simulink model "walkingRobotOptim"  (R2024b)
settings: Solver=ode15s  StartTime=0.0  StopTime=10  EnableMultiTasking=on
PreLoadFcn:
  | robotParameters
  | 
  | % Trajectory sample time
  | tsTraj = 0.01;
  | 
  | % Simulate air drag for stability
  | world_damping = 20; % Translational damping
  | world_rot_damping = 10;  % Rotational damping
  | 
  | % Only run if CAD model has changed on OnShape
  | %run("OnshapeTest\Onshape_Test.m")
  | run("OnshapeTest\Assembly1_DataFile.m")
InitFcn:
  |     % Evaluate the trajectory at the start and halfway points for right and
  |     % left legs, respectively, to get initial conditions and trajectory
  |     % waypoint derivatives
  |     [q_F,hip_der_F,knee_der_F] = createSmoothTrajectory( ...
  |         hip_motion_F,knee_motion_F,gait_period,[0 gait_period/2]);
  |     % Package up the initial conditions, keeping the yaw/roll joints fixed
  |     init_angs_FR = [-q_F(1,1) -q_F(2,1)];
  |     init_angs_FL = [-q_F(1,2) -q_F(2,2)];
  | 
  |     [q_H,hip_der_H,knee_der_H] = createSmoothTrajectory( ...
  |         hip_motion_H,knee_motion_H,gait_period,[0 gait_period/2]);
  |     % Package up the initial conditions, keeping the yaw/roll joints fixed
  |     init_angs_HR = [-q_H(1,1) -q_H(2,1)];
  |     init_angs_HL = [-q_H(1,2) -q_H(2,2)];
values from neighbouring files (symbols this model uses):
  gait_period = 2.5    [optimizedData_06Dec24_1101.mat]
  hip_der = [0, 0.5*( diff(hip(1:end-1)) + diff(hip(2:end)) )/dt, 0]    [createSmoothTrajectory.m]
  hip_motion_F = [-0.788016157275 -1.71688038519 -1.07878801066 0.273318560862 -0.349065850399]    [cheetah_waypoints.mat]    (also in optimizedData_06Dec24_1101.mat = [0.00380771774733 0.00304617419787 0.000761543549467 -0.0045; simulateWalkingRobot.m = deg2rad([params(1:N), params(1)]); walking_waypoints.mat = [-0.617466438509 -0.382533561491 0.182533561491 -0.382533561)
  hip_motion_H = [-0.350287580875 -0.0639663170856 1.07512281923 1.78425009431 0.280474410795]    [cheetah_waypoints.mat]    (also in optimizedData_06Dec24_1101.mat = [-0.0297001984292 0.827036294721 -0.277963395555 0.274155677; simulateWalkingRobot.m = deg2rad([params(2*N+1:3*N), params(2*N+1)]); walking_waypoints.mat = [-0.162257957554 -0.481537983524 -0.286227619971 0.130023561)
  knee_der = [0, 0.5*( diff(knee(1:end-1)) + diff(knee(2:end)) )/dt, 0]    [createSmoothTrajectory.m]
  knee_motion_F = [-0.479791011373 -1.75833195492 -2.37556764489 -1.2809844045 -0.532499954783]    [cheetah_waypoints.mat]    (also in optimizedData_06Dec24_1101.mat = [0.011423153242 0.0144693274399 0.0137077838904 0.0129462403; simulateWalkingRobot.m = deg2rad([params(N+1:2*N), params(N+1)]); walking_waypoints.mat = [0.119729530542 0.911553841048 0.391887203398 0.376829425011)
  knee_motion_H = [0.760789020944 2.09910749137 2.35340196339 1.93007235332 0.791332282854]    [cheetah_waypoints.mat]    (also in optimizedData_06Dec24_1101.mat = [-0.34269459726 -0.132508577607 -0.389148753778 0.1713472986; simulateWalkingRobot.m = deg2rad([params(3*N+1:4*N), params(3*N+1)]); walking_waypoints.mat = [0.397308136111 0.290525222789 0.655140986828 0.257025654272)
  N = numel(params)/4    [simulateWalkingRobot.m]
  traj_times = [0 0.25 0.5 0.75 1]    [cheetah_waypoints.mat]    (also in createSmoothTrajectory.m = linspace(0,period,numPoints); optimizedData_06Dec24_1101.mat = [0 0.5 1 1.5 2 2.5]; simulateWalkingRobot.m = linspace(0,gait_period,N+1); walking_waypoints.mat)
undefined symbols (not defined in the file or in its folder): ankle_der, back_leg_weight, body_weight, gravity, half_leg_weight, hip_der_F, hip_der_H, init_angs_R, knee_der_F, knee_der_H, plane_z, smiData, X, Y, Z
libraries: sm_lib x46, walkingRobotUtils x13, nesl_utility x4, robotcorelib x4, simulink x2
(part 1 of 2)
settings Model: SimulationMode=accelerator  Creator=bkim  LastModifiedBy=Andrew
settings SolverCC: AlgebraicLoopSolver=TrustRegion
settings DataIOCC: ReturnWorkspaceOutputs=off  OutputSaveName=simout  OutputTimes=0:0.01:10
settings OptimizationCC: LifeSpan=inf
settings DebuggingCC: UnconnectedInputMsg=warning  UnconnectedOutputMsg=warning  UnconnectedLineMsg=warning  AllowSymbolicDim=off  PregeneratedLibrarySubsystemCodeDiagnostic=none  SFUnexpectedBacktrackingDiag=warning  SFNoUnconditionalDefaultTransitionDiag=warning  SFExecutionAtInitializationDiag=none  UnitsInconsistencyMsg=none  ArithmeticOperatorsInVariantConditions=warning
settings ModelReferenceCC: EnableRefExpFcnMdlSchedulingChecks=on
settings SFSimCC: SimUseLocalCustomCode=off  CustomCodeUndefinedFunction=UseInterfaceOnly
settings RTWCC: RTWUseLocalCustomCode=off  GPUComputeCapability=3.5
settings CodeAppCC: StateflowObjectComments=on
settings GRTTargetCC: TargetLangStandard=C89/C90 (ANSI)
settings ConfigComp: CovMetricSettings=dw  CovSaveCumulativeToWorkspaceVar=on  CovSaveSingleToWorkspaceVar=on  CovExternalEMLEnable=off  CovSFcnEnable=off
settings SimscapeCC: SimscapeNormalizeSystem=off  SimscapeLogOpenViewer=on  SimscapeLogLimitData=off  SimscapeLogDataHistory=10000
settings ConfigurationSet: Description=SimMechanics 2G
settings DiagnosticsConfigSet: SimMechanicsRigidlyBoundBlock=none
settings ExplorerConfigSet: SimMechanicsOpenEditorOnUpdate=off  InternalSimMechanicsExplorerSettings="<ExplorerConfiguration><canonicalview>default</canonicalview><AnimationSetting><BasePlaybackSpeed>1.0</BasePlaybackSpeed><PlaybackSpeedFactor>1.0</PlaybackSpeedFactor></AnimationSetting><TilePanel><TileInfo><Tiles Columns=\"1\" Count=\"1\" Rows=\"1\"><Column Weight=\"1\"/><Row Weight=\"1\"/><Tile Height=\"1\" Width=\"1\" X=\"0\" Y=\"0\"/></Tiles></TileInfo><SceneInfo><SceneViewer><BGColor><R>0.60000002384185791</R><G>0.60000002384185791</G><B>0.60000002384185791</B></BGColor><Camera><DoPerspective>off</DoPerspective><Position><X>-6.96629667239135308</X><Y>24.6054722866086557</Y><Z>5.12968018743748999</Z></Position><Center><X>2.4732135105562727</X><Y>-3.90012739093662164</Y><Z>-2.29509835736230228</Z></Center><Up><X>0.317576681516579584</X><Y>-0.139145800878009762</Y><Z>0.937967748621952424</Z></Up><ViewLimDist>1</ViewLimDist><YLim>3.00115752214017162</YLim><XLim>3.84407522125978751</XLim></Camera></SceneViewer></SceneInfo></TilePanel><MechEditorPanel><Cameras/><GfxPanelCameraMap/><VideoCreator><PlaybackSpeedRatio>1.0</PlaybackSpeedRatio><FrameRate>30</FrameRate><VideoFormat>Motion JPEG AVI</VideoFormat><FrameSize>auto</FrameSize></VideoCreator></MechEditorPanel></ExplorerConfiguration>"

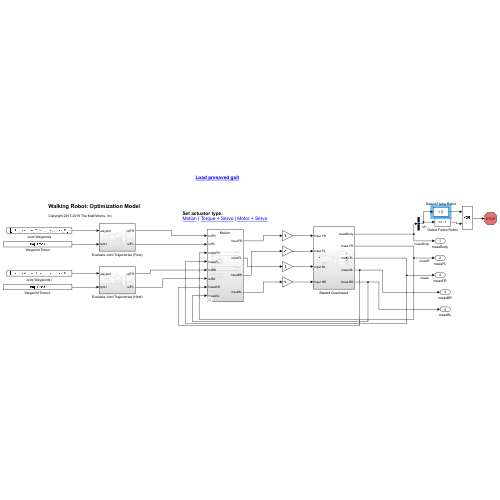
[thumbnail: Simulink's stored preview of the top-level diagram]
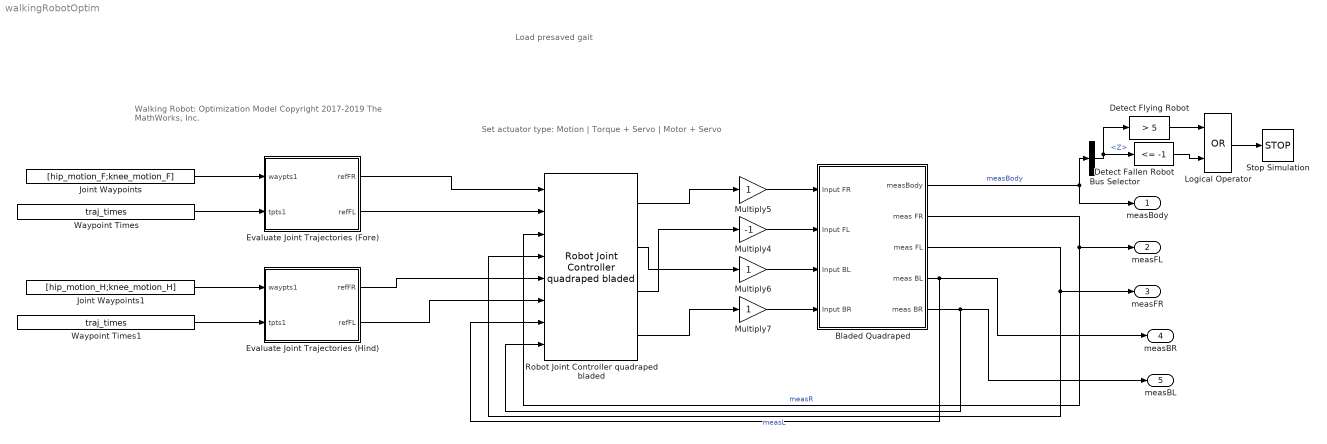
== system walkingRobotOptim ==
  note: Load presaved gait
  note: Walking Robot: Optimization Model
      |
      | Copyright 2017-2019 The MathWorks, Inc.
  note: Set actuator type:
      | Motion | Torque + Servo | Motor + Servo
  Bladed Quadraped : Subsystem
  Bus Selector : BusSelector  OutputSignals=Z
  Detect Fallen Robot : simulink/Logic and Bit Operations/Compare To Constant  relop=<=  const=-1  OutDataTypeStr=boolean
  Detect Flying Robot : simulink/Logic and Bit Operations/Compare To Constant  relop=>  const=5  OutDataTypeStr=boolean
  Evaluate Joint Trajectories (Fore) : Subsystem
  Evaluate Joint Trajectories (Hind) : Subsystem
  Joint Waypoints : Constant  Value=[hip_motion_F;knee_motion_F]
  Joint Waypoints1 : Constant  Value=[hip_motion_H;knee_motion_H]
  Logical Operator : Logic  Operator=OR  AllPortsSameDT=off  OutDataTypeStr=boolean
  Multiply4 : Gain  Gain=-1
  Multiply5 : Gain
  Multiply6 : Gain
  Multiply7 : Gain
  Robot Joint Controller quadraped bladed : walkingRobotUtils/Robot Joint Controller quadraped bladed  SystemSampleTime=-1  VariantActivationTime=update diagram  AllowFlexibleInterface=on  Latency=0  AutoFrameSizeCalculation=off
  Stop Simulation : Stop
  Waypoint Times : Constant  Value=traj_times
  Waypoint Times1 : Constant  Value=traj_times
  measBody : Outport  VectorParamsAs1DForOutWhenUnconnected=off
  measFL : Outport  Port=2  VectorParamsAs1DForOutWhenUnconnected=off
  measFR : Outport  Port=3  VectorParamsAs1DForOutWhenUnconnected=off
  measBR : Outport  Port=4  VectorParamsAs1DForOutWhenUnconnected=off
  measBL : Outport  Port=5  VectorParamsAs1DForOutWhenUnconnected=off
  wires:
  Bladed Quadraped/3(meas FL) -> Robot Joint Controller quadraped bladed/4, measFR/1  "measL"
  Bladed Quadraped/2(meas FR) -> Robot Joint Controller quadraped bladed/3, measFL/1  "measR"
  Bladed Quadraped/1(measBody) -> measBody/1, Bus Selector/1  "measBody"
  Bus Selector/1 -> Detect Flying Robot/1, Detect Fallen Robot/1  "<Z>"
  Detect Fallen Robot/1 -> Logical Operator/2
  Logical Operator/1 -> Stop Simulation/1
  Detect Flying Robot/1 -> Logical Operator/1
  Bladed Quadraped/4(meas BL) -> Robot Joint Controller quadraped bladed/7, measBR/1
  Bladed Quadraped/5(meas BR) -> Robot Joint Controller quadraped bladed/8, measBL/1
  Joint Waypoints/1 -> Evaluate Joint Trajectories (Fore)/1(waypts1)
  Evaluate Joint Trajectories (Fore)/1(refFR) -> Robot Joint Controller quadraped bladed/1
  Waypoint Times/1 -> Evaluate Joint Trajectories (Fore)/2(tpts1)
  Robot Joint Controller quadraped bladed/1 -> Multiply5/1
  Multiply6/1 -> Bladed Quadraped/3(Input BL)
  Robot Joint Controller quadraped bladed/4 -> Multiply7/1
  Multiply5/1 -> Bladed Quadraped/1(Input FR)
  Multiply7/1 -> Bladed Quadraped/4(Input BR)
  Robot Joint Controller quadraped bladed/2 -> Multiply6/1
  Multiply4/1 -> Bladed Quadraped/2(Input FL)
  Robot Joint Controller quadraped bladed/3 -> Multiply4/1
  Evaluate Joint Trajectories (Fore)/2(refFL) -> Robot Joint Controller quadraped bladed/2
  Evaluate Joint Trajectories (Hind)/1(refFR) -> Robot Joint Controller quadraped bladed/5
  Waypoint Times1/1 -> Evaluate Joint Trajectories (Hind)/2(tpts1)
  Joint Waypoints1/1 -> Evaluate Joint Trajectories (Hind)/1(waypts1)
  Evaluate Joint Trajectories (Hind)/2(refFL) -> Robot Joint Controller quadraped bladed/6

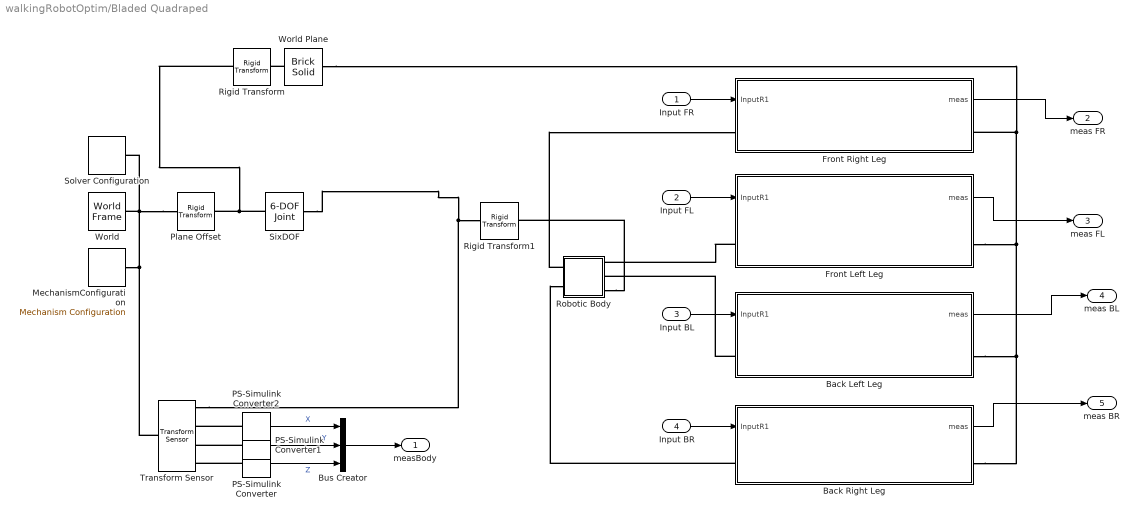
== system walkingRobotOptim/Bladed Quadraped ==
  Input FR : Inport
  Input FL : Inport  Port=2
  Input BL : Inport  Port=3
  Input BR : Inport  Port=4
  Back Left Leg : Subsystem
  Back Right Leg : Subsystem
  Bus Creator : BusCreator  Inputs=3
  Front Left Leg : Subsystem
  Front Right Leg : Subsystem
  MechanismConfiguration : sm_lib/Utilities/Mechanism Configuration  UniformGravity=Constant  GravityVector="[0 0  -gravity]"  GravityVectorUnits=m/s^2  LinearizationDelta=0.001  JointModeTransitionNonlinearIterations=2
  PS-Simulink Converter : nesl_utility/PS-Simulink Converter  PhysicalDomain=network_engine_domain  SubClassName=ps_output  LeftPortType=input  RightPortType=output  PseudoPeriodic=off  Frequencies=[]  VectorFormat=1-D array  Unit=m  AffineConversion=off
  PS-Simulink Converter1 : nesl_utility/PS-Simulink Converter  PhysicalDomain=network_engine_domain  SubClassName=ps_output  LeftPortType=input  RightPortType=output  PseudoPeriodic=off  Frequencies=[]  VectorFormat=1-D array  Unit=m  AffineConversion=off
  PS-Simulink Converter2 : nesl_utility/PS-Simulink Converter  PhysicalDomain=network_engine_domain  SubClassName=ps_output  LeftPortType=input  RightPortType=output  PseudoPeriodic=off  Frequencies=[]  VectorFormat=1-D array  Unit=m  AffineConversion=off
  Plane Offset : sm_lib/Frames and Transforms/Rigid Transform  RotationMethod=ArbitraryAxis  FollAlignAxisA=+X  BaseAlignAxisA=+Y  FollAlignAxisB=+Y  BaseAlignAxisB=+Z  RotationStandardAxis=+Z  RotationAngle=smiData.RigidTransform(17).angle  RotationAngleUnits=rad  RotationArbitraryAxis=smiData.RigidTransform(17).axis  RotationSequenceAxes=FollowerAxes  RotationSequence=XYX  RotationSequenceAngles=[0 0 0]  RotationSequenceAnglesUnits=deg  RotationMatrix=[1 0 0;0 1 0;0 0 1]  Quaternion=[1 0 0 0]  TranslationMethod=Cartesian  TranslationCartesianOffset=smiData.RigidTransform(17).translation  TranslationCartesianOffsetUnits=mm  TranslationStandardAxis=+Z  TranslationStandardOffset=0  TranslationStandardOffsetUnits=m  TranslationROffset=0  TranslationROffsetUnits=m  TranslationThetaOffset=0  TranslationThetaOffsetUnits=deg  TranslationZOffset=0  TranslationZOffsetUnits=m
  Rigid Transform : sm_lib/Frames and Transforms/Rigid Transform  RotationMethod=StandardAxis  FollAlignAxisA=+X  BaseAlignAxisA=+Y  FollAlignAxisB=+Y  BaseAlignAxisB=+Z  RotationStandardAxis=+Z  RotationAngle=90  RotationAngleUnits=deg  RotationArbitraryAxis=[0 0 1]  RotationSequenceAxes=FollowerAxes  RotationSequence=XYX  RotationSequenceAngles=[0 0 0]  RotationSequenceAnglesUnits=deg  RotationMatrix=[1 0 0;0 1 0;0 0 1]  Quaternion=[1 0 0 0]  TranslationMethod=StandardAxis  TranslationCartesianOffset=[0 0 0]  TranslationCartesianOffsetUnits=m  TranslationStandardAxis=+Z  TranslationStandardOffset=1  TranslationStandardOffsetUnits=m  TranslationROffset=0  TranslationROffsetUnits=m  TranslationThetaOffset=0  TranslationThetaOffsetUnits=deg  TranslationZOffset=0  TranslationZOffsetUnits=m
  Rigid Transform1 : sm_lib/Frames and Transforms/Rigid Transform  RotationMethod=StandardAxis  FollAlignAxisA=+X  BaseAlignAxisA=+Y  FollAlignAxisB=+Y  BaseAlignAxisB=+Z  RotationStandardAxis=-X  RotationAngle=180  RotationAngleUnits=deg  RotationArbitraryAxis=[0 0 1]  RotationSequenceAxes=FollowerAxes  RotationSequence=XYX  RotationSequenceAngles=[0 0 0]  RotationSequenceAnglesUnits=deg  RotationMatrix=[1 0 0;0 1 0;0 0 1]  Quaternion=[1 0 0 0]  TranslationMethod=None  TranslationCartesianOffset=[0 0 0]  TranslationCartesianOffsetUnits=m  TranslationStandardAxis=+Z  TranslationStandardOffset=1.5  TranslationStandardOffsetUnits=m  TranslationROffset=0  TranslationROffsetUnits=m  TranslationThetaOffset=0  TranslationThetaOffsetUnits=deg  TranslationZOffset=0  TranslationZOffsetUnits=m
  Robotic Body : Subsystem
  SixDOF : sm_lib/Joints/6-DOF Joint  JointMode=Normal  CompositeWrenchDir=FollowerOnBase  CompositeWrenchFrame=BaseFrame  SenseConstraintForce=off  SenseConstraintTorque=off  SenseTotalForce=off  SenseTotalTorque=off  PxPositionTargetSpecify=off  PxPositionTargetPriority=High  PxPositionTargetValue=0  PxPositionTargetValueUnits=m  PxVelocityTargetSpecify=off  PxVelocityTargetPriority=High  PxVelocityTargetValue=0  PxVelocityTargetValueUnits=m/s  PxEquilibriumPosition=0  PxEquilibriumPositionUnits=m  PxSpringStiffness=0  PxSpringStiffnessUnits=N/m  PxDampingCoefficient=0  PxDampingCoefficientUnits=N/(m/s)  PxLowerLimitSpecify=off  PxLowerLimitBound=-1  PxLowerLimitBoundUnits=m  PxLowerLimitStiffness=1e6  PxLowerLimitStiffnessUnits=N/m  PxLowerLimitDamping=1e3  PxLowerLimitDampingUnits=N/(m/s)  PxLowerLimitTransitionRegionWidth=1e-4  PxLowerLimitTransitionRegionWidthUnits=m  PxUpperLimitSpecify=off  PxUpperLimitBound=1  PxUpperLimitBoundUnits=m  PxUpperLimitStiffness=1e6  PxUpperLimitStiffnessUnits=N/m  PxUpperLimitDamping=1e3  PxUpperLimitDampingUnits=N/(m/s)  PxUpperLimitTransitionRegionWidth=1e-4  PxUpperLimitTransitionRegionWidthUnits=m  PxTorqueActuationMode=NoTorque  PxMotionActuationMode=ComputedMotion  PxSensePosition=off  PxSenseVelocity=off  PxSenseAcceleration=off  PxSenseTorqueForce=off  PxSenseLowerLimitTorqueForce=off  PxSenseUpperLimitTorqueForce=off  PyPositionTargetSpecify=off  PyPositionTargetPriority=High  PyPositionTargetValue=0  PyPositionTargetValueUnits=m  PyVelocityTargetSpecify=off  PyVelocityTargetPriority=High  PyVelocityTargetValue=0  PyVelocityTargetValueUnits=m/s  PyEquilibriumPosition=0  PyEquilibriumPositionUnits=m  PySpringStiffness=0  PySpringStiffnessUnits=N/m  PyDampingCoefficient=0  PyDampingCoefficientUnits=N/(m/s)  PyLowerLimitSpecify=off  PyLowerLimitBound=-1  PyLowerLimitBoundUnits=m  PyLowerLimitStiffness=1e6  PyLowerLimitStiffnessUnits=N/m  PyLowerLimitDamping=1e3  PyLowerLimitDampingUnits=N/(m/s)  PyLowerLimitTransitionRegionWidth=1e-4  PyLowerLimitTransitionRegionWidthUnits=m  PyUpperLimitSpecify=off  PyUpperLimitBound=1  PyUpperLimitBoundUnits=m  PyUpperLimitStiffness=1e6  PyUpperLimitStiffnessUnits=N/m  PyUpperLimitDamping=1e3  PyUpperLimitDampingUnits=N/(m/s)  PyUpperLimitTransitionRegionWidth=1e-4  PyUpperLimitTransitionRegionWidthUnits=m  PyTorqueActuationMode=NoTorque  PyMotionActuationMode=ComputedMotion  PySensePosition=off  PySenseVelocity=off  PySenseAcceleration=off  PySenseTorqueForce=off  PySenseLowerLimitTorqueForce=off  PySenseUpperLimitTorqueForce=off  PzPositionTargetSpecify=off  PzPositionTargetPriority=High  PzPositionTargetValue=0  PzPositionTargetValueUnits=m  PzVelocityTargetSpecify=off  PzVelocityTargetPriority=High  PzVelocityTargetValue=0  PzVelocityTargetValueUnits=m/s  PzEquilibriumPosition=0  PzEquilibriumPositionUnits=m  PzSpringStiffness=0  PzSpringStiffnessUnits=N/m  PzDampingCoefficient=0  PzDampingCoefficientUnits=N/(m/s)  PzLowerLimitSpecify=off  PzLowerLimitBound=-1  PzLowerLimitBoundUnits=m  PzLowerLimitStiffness=1e6  PzLowerLimitStiffnessUnits=N/m  PzLowerLimitDamping=1e3  PzLowerLimitDampingUnits=N/(m/s)  PzLowerLimitTransitionRegionWidth=1e-4  PzLowerLimitTransitionRegionWidthUnits=m  PzUpperLimitSpecify=off  PzUpperLimitBound=1  PzUpperLimitBoundUnits=m  PzUpperLimitStiffness=1e6  PzUpperLimitStiffnessUnits=N/m  PzUpperLimitDamping=1e3  PzUpperLimitDampingUnits=N/(m/s)  PzUpperLimitTransitionRegionWidth=1e-4  PzUpperLimitTransitionRegionWidthUnits=m  PzTorqueActuationMode=NoTorque  PzMotionActuationMode=ComputedMotion  PzSensePosition=off  PzSenseVelocity=off  PzSenseAcceleration=off  PzSenseTorqueForce=off  PzSenseLowerLimitTorqueForce=off  PzSenseUpperLimitTorqueForce=off  SphPositionTargetSpecify=off  SphPositionTargetPriority=High  SphPositionTargetRotationMethod=None  SphPositionTargetFollAlignAxisA=+X  SphPositionTargetBaseAlignAxisA=+Y  SphPositionTargetFollAlignAxisB=+Y  SphPositionTargetBaseAlignAxisB=+Z  SphPositionTargetRotationStandardAxis=+Z  SphPositionTargetRotationAngle=0  SphPositionTargetRotationAngleUnits=deg  SphPositionTargetRotationArbitraryAxis=[0 0 1]  SphPositionTargetRotationSequenceAxes=FollowerAxes  SphPositionTargetRotationSequence=XYX  SphPositionTargetRotationSequenceAngles=[0 0 0]  SphPositionTargetRotationSequenceAnglesUnits=deg  SphPositionTargetRotationMatrix=[1 0 0;0 1 0;0 0 1]  SphPositionTargetQuaternion=[1 0 0 0]  SphVelocityTargetSpecify=off  SphVelocityTargetPriority=High  SphVelocityTargetValue=[0 0 0]  SphVelocityTargetValueUnits=deg/s  SphVelocityTargetInFollowerFrame=on  SphEqPosRotationMethod=None  SphEqPosFollAlignAxisA=+X  SphEqPosBaseAlignAxisA=+Y  SphEqPosFollAlignAxisB=+Y  SphEqPosBaseAlignAxisB=+Z  SphEqPosRotationStandardAxis=+Z  SphEqPosRotationAngle=0  SphEqPosRotationAngleUnits=deg  SphEqPosRotationArbitraryAxis=[0 0 1]  SphEqPosRotationSequenceAxes=FollowerAxes  SphEqPosRotationSequence=XYX  SphEqPosRotationSequenceAngles=[0 0 0]  SphEqPosRotationSequenceAnglesUnits=deg  SphEqPosRotationMatrix=[1 0 0;0 1 0;0 0 1]  SphEqPosQuaternion=[1 0 0 0]  SphSpringStiffness=0  SphSpringStiffnessUnits=N*m/deg  SphDampingCoefficient=0  SphDampingCoefficientUnits=N*m/(deg/s)  SphLowerLimitSpecify=off  SphLowerLimitBound=15  SphLowerLimitBoundUnits=deg  SphLowerLimitStiffness=1e4  SphLowerLimitStiffnessUnits=N*m/deg  SphLowerLimitDamping=10  SphLowerLimitDampingUnits=N*m/(deg/s)  SphLowerLimitTransitionRegionWidth=0.1  SphLowerLimitTransitionRegionWidthUnits=deg  SphUpperLimitSpecify=off  SphUpperLimitBound=45  SphUpperLimitBoundUnits=deg  SphUpperLimitStiffness=1e4  SphUpperLimitStiffnessUnits=N*m/deg  SphUpperLimitDamping=10  SphUpperLimitDampingUnits=N*m/(deg/s)  SphUpperLimitTransitionRegionWidth=0.1  SphUpperLimitTransitionRegionWidthUnits=deg  SphTorqueActuationMode=NoTorque  SphActuateTorqueX=off  SphActuateTorqueY=off  SphActuateTorqueZ=off  SphActuateTorque=off  SphActuationFrame=BaseFrame  SphSensePosition=off  SphSenseVelocityX=off  SphSenseVelocityY=off  SphSenseVelocityZ=off  SphSenseVelocity=off  SphSenseAccelerationX=off  SphSenseAccelerationY=off  SphSenseAccelerationZ=off  SphSenseAcceleration=off  SphSenseLowerLimitTorqueMag=off  SphSenseUpperLimitTorqueMag=off  SphSensingFrame=FollowerFrame
  Solver Configuration : nesl_utility/Solver Configuration  PhysicalDomain=network_engine_domain  SubClassName=solver  LeftPortType=input  RightPortType=generic  Tones=[]  Harmonics=[]  SimulateNoise=off  Profile=off  UseLocalSampling=off  EnableSwitchedLinearOptims=on  FrequencyDomain=off  UseCCode=off  RelTol=0.001  AbsTol=0.001  MinStep=1e-09  ToWorkspace=off  RevertToSquareIcSolve=off  NumHomotopyIterations=100  PhasorMode=off  PhasorModeNumHarmonics=1  ConsistencySolver=NEWTON_XTOL_AFTER_FTOL  IndexReductionMethod=DerivativeReplacement  DoDC=off  ResidualTolerance=1e-09  ConsistencyTolSource=GLOBAL  ConsistencyAbsTol=0.001  ConsistencyRelTol=0.001  ConsistencyTolFactor=0.001  UseLocalSolver=off  LocalSolverChoice=NE_BACKWARD_EULER_ADVANCER  ResolveIndetEquations=on  FunctionEvalNumThread=1  LocalSolverSampleTime=0.001  DoFixedCost=off  MaxNonlinIter=3  MaxModeIter=2  ComputeImpulses=off  ImpulseIterations=2  LinearAlgebra=auto  LinearAlgebraNumThread=0  EquationFormulation=NE_TIME_EF  DelaysMemoryBudget=1024  AutomaticFiltering=on  FilteringTimeConstant=0.001  PartitionStorageMethod=AS_NEEDED  PartitionMemoryBudget=1024  PartitionMethod=ROBUST  MultibodyUseLocalSolver=off  MultibodyLocalSolverChoice=ODE1  MultibodyLocalSolverSampleTime=0.001
  Transform Sensor : sm_lib/Frames and Transforms/Transform Sensor  MeasurementFrame=World  RotationSequence=XYX  SenseAngle=off  SenseAxis=off  SenseQ=off  SenseR=off  SenseRotationSequence=off  SenseOmegaX=off  SenseOmegaY=off  SenseOmegaZ=off  SenseOmega=off  SenseQDot=off  SenseRDot=off  SenseRotationSequenceDot=off  SenseAlphaX=off  SenseAlphaY=off  SenseAlphaZ=off  SenseAlpha=off  SenseQDDot=off  SenseRDDot=off  SenseX=on  SenseY=on  SenseZ=on  SenseXYZ=off  SenseRad=off  SenseAzim=off  SenseDist=off  SenseInc=off  SenseXDot=off  SenseYDot=off  SenseZDot=off  SenseXYZDot=off  SenseRadDot=off  SenseAzimDot=off  SenseDistDot=off  SenseIncDot=off  SenseXDDot=off  SenseYDDot=off  SenseZDDot=off  SenseXYZDDot=off  SenseRadDDot=off  SenseAzimDDot=off  SenseDistDDot=off  SenseIncDDot=off
  World : sm_lib/Frames and Transforms/World Frame
  World Plane : sm_lib/Body Elements/Brick Solid  BrickDimensions=[100 100 plane_z]  BrickDimensionsUnits=m  ExportEntireGeometry=on  InertiaType=CalculateFromGeometry  BasedOnType=Density  Density=1000  DensityUnits=kg/(m^3)  Mass=1  MassUnits=kg  CenterOfMass=[0 0 0]  CenterOfMassUnits=m  MomentsOfInertia=[1 1 1]  MomentsOfInertiaUnits=kg*m^2  ProductsOfInertia=[0 0 0]  ProductsOfInertiaUnits=kg*m^2  GraphicType=FromGeometry  MarkerShape=Sphere  MarkerSize=10  GraphicVisPropType=SimpleVisualProperties  GraphicDiffuseColor=[0.6353 0.07843 0.1843]  GraphicOpacity=1  GraphicSpecularColor=[0.5 0.5 0.5 1.0]  GraphicAmbientColor=[0.15 0.15 0.15 1.0]  GraphicEmissiveColor=[0.0 0.0 0.0 1.0]  GraphicShininess=75  DoExposeReferenceFrame=on  SerializedFrames=<Frames/>
  measBody : Outport  VectorParamsAs1DForOutWhenUnconnected=off
  meas FR : Outport  Port=2  VectorParamsAs1DForOutWhenUnconnected=off
  meas FL : Outport  Port=3  VectorParamsAs1DForOutWhenUnconnected=off
  meas BL : Outport  Port=4  VectorParamsAs1DForOutWhenUnconnected=off
  meas BR : Outport  Port=5  VectorParamsAs1DForOutWhenUnconnected=off
  wires:
  PS-Simulink Converter1/1 -> Bus Creator/2  "Y"
  Bus Creator/1 -> measBody/1
  PS-Simulink Converter2/1 -> Bus Creator/1  "X"
  PS-Simulink Converter/1 -> Bus Creator/3  "Z"
  Input BR/1 -> Back Right Leg/1(InputR1)
  Front Right Leg/1(meas) -> meas FR/1
  Front Left Leg/1(meas) -> meas FL/1
  Back Left Leg/1(meas) -> meas BL/1
  Back Right Leg/1(meas) -> meas BR/1
  Input FL/1 -> Front Left Leg/1(InputR1)
  Input FR/1 -> Front Right Leg/1(InputR1)
  Input BL/1 -> Back Left Leg/1(InputR1)
  connections:
  Plane Offset/LConn1 -- Transform Sensor/LConn1 -- MechanismConfiguration/RConn1 -- Solver Configuration/RConn1 -- World/RConn1
  Back Left Leg/LConn1 -- Robotic Body/RConn2
  SixDOF/RConn1 -- Transform Sensor/RConn1 -- Rigid Transform1/LConn1
  Back Right Leg/LConn1 -- Robotic Body/LConn2
  Front Left Leg/LConn1 -- Robotic Body/RConn1
  PS-Simulink Converter1/LConn1 -- Transform Sensor/RConn3
  PS-Simulink Converter2/LConn1 -- Transform Sensor/RConn2
  PS-Simulink Converter/LConn1 -- Transform Sensor/RConn4
  World Plane/LConn1 -- Back Right Leg/RConn1 -- Back Left Leg/RConn1 -- Front Left Leg/RConn1 -- Front Right Leg/RConn1
  World Plane/RConn1 -- Rigid Transform/RConn1
  Plane Offset/RConn1 -- Rigid Transform/LConn1 -- SixDOF/LConn1
  Robotic Body/LConn1 -- Front Right Leg/LConn1
  Robotic Body/RConn3 -- Rigid Transform1/RConn1

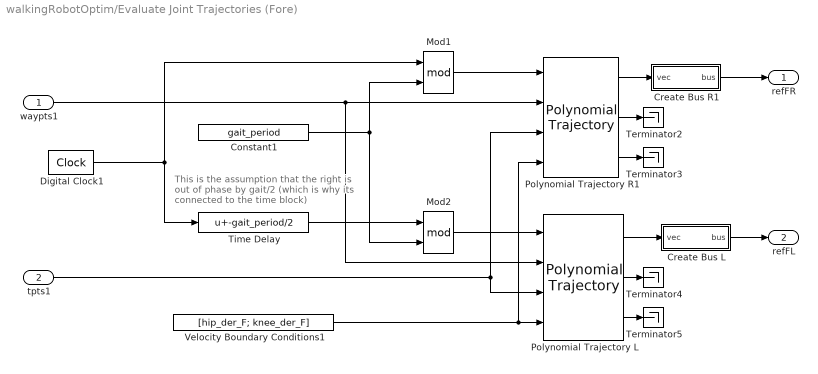
== system walkingRobotOptim/Evaluate Joint Trajectories (Fore) ==
  note: This is the assumption that the right is out of phase by gait/2 (which is why its connected to the time block)
  waypts1 : Inport
  tpts1 : Inport  Port=2
  Constant1 : Constant  Value=gait_period
  Create Bus L : Subsystem
  Create Bus R1 : Subsystem
  Digital Clock1 : DigitalClock  SampleTime=.01
  Mod1 : Math  Operator=mod
  Mod2 : Math  Operator=mod
  Polynomial Trajectory L : robotcorelib/Polynomial Trajectory  WaypointSource=External  Waypoints=[ 0, 2, 1, 5, 0; -1, 3, 1, 4, 4 ]  TimePoints=time  TimeInterval=[ 1, 4 ]  Method=Cubic Polynomial  ParameterSource=External  VelocityBoundaryCondition=[hip_der; knee_der; ankle_der]  AccelerationBoundaryCondition=zeros( 2, 5 )  SimulateUsing=Code generation
  Polynomial Trajectory R1 : robotcorelib/Polynomial Trajectory  WaypointSource=External  Waypoints=[ 0, 2, 1, 5, 0; -1, 3, 1, 4, 4 ]  TimePoints=time  TimeInterval=[ 1, 4 ]  Method=Cubic Polynomial  ParameterSource=External  VelocityBoundaryCondition=[hip_der; knee_der; ankle_der]  AccelerationBoundaryCondition=zeros( 2, 5 )  SimulateUsing=Code generation
  Terminator{2..5} (4 alike) : Terminator
  Time Delay : Bias  Bias=-gait_period/2  SaturateOnIntegerOverflow=off
  Velocity Boundary Conditions1 : Constant  Value=[hip_der_F; knee_der_F]
  refFR : Outport
  refFL : Outport  Port=2
  wires:
  Polynomial Trajectory L/3 -> Terminator5/1
  Velocity Boundary Conditions1/1 -> Polynomial Trajectory R1/4, Polynomial Trajectory L/4
  Create Bus L/1(bus) -> refFL/1
  Mod2/1 -> Polynomial Trajectory L/1
  Digital Clock1/1 -> Time Delay/1, Mod1/1
  Polynomial Trajectory R1/2 -> Terminator2/1
  tpts1/1 -> Polynomial Trajectory L/3, Polynomial Trajectory R1/3
  Polynomial Trajectory R1/3 -> Terminator3/1
  Polynomial Trajectory L/2 -> Terminator4/1
  Polynomial Trajectory R1/1 -> Create Bus R1/1(vec)
  waypts1/1 -> Polynomial Trajectory L/2, Polynomial Trajectory R1/2
  Mod1/1 -> Polynomial Trajectory R1/1
  Constant1/1 -> Mod1/2, Mod2/2
  Polynomial Trajectory L/1 -> Create Bus L/1(vec)
  Time Delay/1 -> Mod2/1
  Create Bus R1/1(bus) -> refFR/1

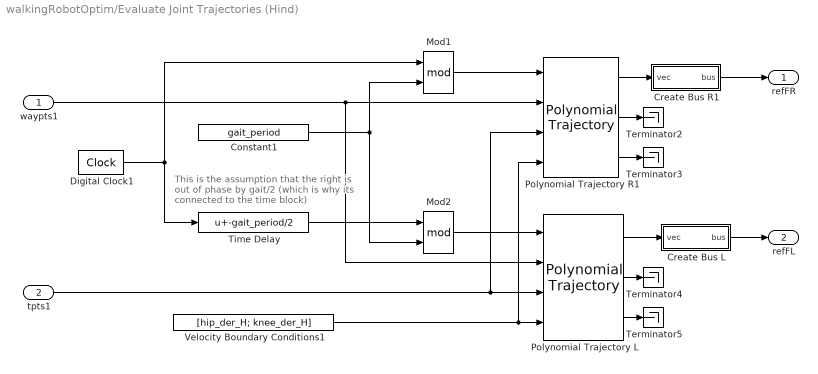
== system walkingRobotOptim/Evaluate Joint Trajectories (Hind) ==
  note: This is the assumption that the right is out of phase by gait/2 (which is why its connected to the time block)
  waypts1 : Inport
  tpts1 : Inport  Port=2
  Constant1 : Constant  Value=gait_period
  Create Bus L : Subsystem
  Create Bus R1 : Subsystem
  Digital Clock1 : DigitalClock  SampleTime=.01
  Mod1 : Math  Operator=mod
  Mod2 : Math  Operator=mod
  Polynomial Trajectory L : robotcorelib/Polynomial Trajectory  WaypointSource=External  Waypoints=[ 0, 2, 1, 5, 0; -1, 3, 1, 4, 4 ]  TimePoints=time  TimeInterval=[ 1, 4 ]  Method=Cubic Polynomial  ParameterSource=External  VelocityBoundaryCondition=[hip_der; knee_der; ankle_der]  AccelerationBoundaryCondition=zeros( 2, 5 )  SimulateUsing=Code generation
  Polynomial Trajectory R1 : robotcorelib/Polynomial Trajectory  WaypointSource=External  Waypoints=[ 0, 2, 1, 5, 0; -1, 3, 1, 4, 4 ]  TimePoints=time  TimeInterval=[ 1, 4 ]  Method=Cubic Polynomial  ParameterSource=External  VelocityBoundaryCondition=[hip_der; knee_der; ankle_der]  AccelerationBoundaryCondition=zeros( 2, 5 )  SimulateUsing=Code generation
  Terminator{2..5} (4 alike) : Terminator
  Time Delay : Bias  Bias=-gait_period/2  SaturateOnIntegerOverflow=off
  Velocity Boundary Conditions1 : Constant  Value=[hip_der_H; knee_der_H]
  refFR : Outport
  refFL : Outport  Port=2
  wires:
  Polynomial Trajectory L/3 -> Terminator5/1
  Velocity Boundary Conditions1/1 -> Polynomial Trajectory R1/4, Polynomial Trajectory L/4
  Create Bus L/1(bus) -> refFL/1
  Mod2/1 -> Polynomial Trajectory L/1
  Digital Clock1/1 -> Time Delay/1, Mod1/1
  Polynomial Trajectory R1/2 -> Terminator2/1
  tpts1/1 -> Polynomial Trajectory R1/3, Polynomial Trajectory L/3
  Polynomial Trajectory R1/3 -> Terminator3/1
  Polynomial Trajectory L/2 -> Terminator4/1
  Polynomial Trajectory R1/1 -> Create Bus R1/1(vec)
  waypts1/1 -> Polynomial Trajectory L/2, Polynomial Trajectory R1/2
  Mod1/1 -> Polynomial Trajectory R1/1
  Constant1/1 -> Mod1/2, Mod2/2
  Polynomial Trajectory L/1 -> Create Bus L/1(vec)
  Time Delay/1 -> Mod2/1
  Create Bus R1/1(bus) -> refFR/1

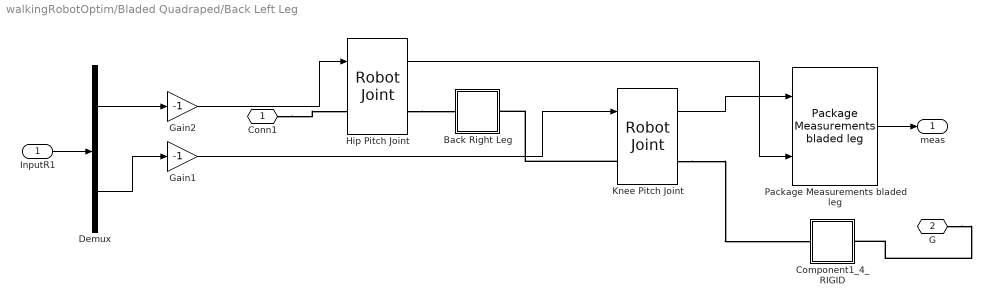
== system walkingRobotOptim/Bladed Quadraped/Back Left Leg ==
  InputR1 : Inport
  Back Right Leg : Subsystem
  Component1_4_RIGID : Subsystem
  Demux : Demux  Outputs=2
  Gain1 : Gain  Gain=-1
  Gain2 : Gain  Gain=-1
  Hip Pitch Joint : walkingRobotUtils/Robot Joint  jointDamping=joint_damping  initAngle=init_angs_HL(1)  upperLimit=pi/2  lowerLimit=-pi/2  limitK=1000  limitD=100
  Knee Pitch Joint : walkingRobotUtils/Robot Joint  jointDamping=joint_damping  initAngle=init_angs_HL(2)  upperLimit=pi/2  lowerLimit=-pi/2  limitK=1000  limitD=100
  Package Measurements bladed leg : walkingRobotUtils/Package Measurements bladed leg  SystemSampleTime=-1  VariantActivationTime=update diagram  AllowFlexibleInterface=on  Latency=0  AutoFrameSizeCalculation=off
  Conn1 : PMIOPort  Side=Left
  G : PMIOPort  Port=2  Side=Right
  meas : Outport  VectorParamsAs1DForOutWhenUnconnected=off
  wires:
  InputR1/1 -> Demux/1
  Gain1/1 -> Knee Pitch Joint/1
  Demux/2 -> Gain1/1
  Demux/1 -> Gain2/1
  Gain2/1 -> Hip Pitch Joint/1
  Hip Pitch Joint/1 -> Package Measurements bladed leg/2
  Knee Pitch Joint/1 -> Package Measurements bladed leg/1
  Package Measurements bladed leg/1 -> meas/1
  connections:
  Conn1/RConn1 -- Hip Pitch Joint/LConn1
  Knee Pitch Joint/RConn1 -- Component1_4_RIGID/LConn1
  G/RConn1 -- Component1_4_RIGID/RConn1
  Hip Pitch Joint/RConn1 -- Back Right Leg/LConn1
  Knee Pitch Joint/LConn1 -- Back Right Leg/RConn1

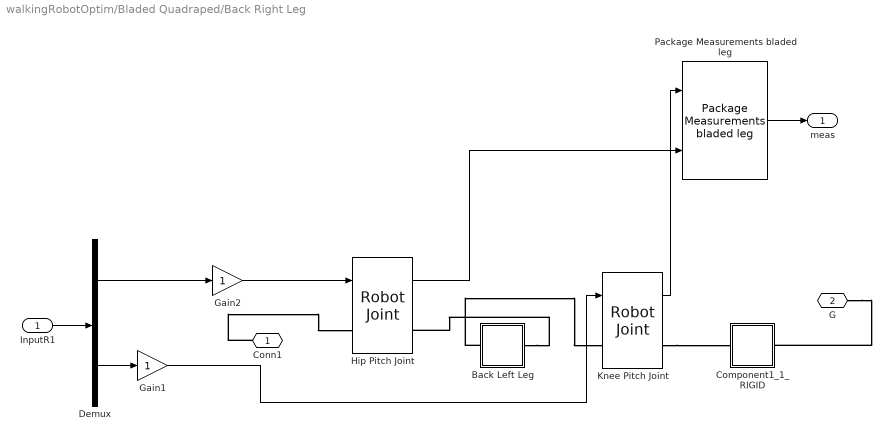
== system walkingRobotOptim/Bladed Quadraped/Back Right Leg ==
  InputR1 : Inport
  Back Left Leg : Subsystem
  Component1_1_RIGID : Subsystem
  Demux : Demux  Outputs=2
  Gain1 : Gain
  Gain2 : Gain
  Hip Pitch Joint : walkingRobotUtils/Robot Joint  jointDamping=joint_damping  initAngle=init_angs_HR(1)  upperLimit=pi/2  lowerLimit=-pi/2  limitK=1000  limitD=100
  Knee Pitch Joint : walkingRobotUtils/Robot Joint  jointDamping=joint_damping  initAngle=init_angs_HR(1)  upperLimit=pi/2  lowerLimit=-pi/2  limitK=1000  limitD=100
  Package Measurements bladed leg : walkingRobotUtils/Package Measurements bladed leg  SystemSampleTime=-1  VariantActivationTime=update diagram  AllowFlexibleInterface=on  Latency=0  AutoFrameSizeCalculation=off
  Conn1 : PMIOPort  Side=Left
  G : PMIOPort  Port=2  Side=Right
  meas : Outport  VectorParamsAs1DForOutWhenUnconnected=off
  wires:
  InputR1/1 -> Demux/1
  Demux/1 -> Gain2/1
  Demux/2 -> Gain1/1
  Hip Pitch Joint/1 -> Package Measurements bladed leg/2
  Package Measurements bladed leg/1 -> meas/1
  Knee Pitch Joint/1 -> Package Measurements bladed leg/1
  Gain2/1 -> Hip Pitch Joint/1
  Gain1/1 -> Knee Pitch Joint/1
  connections:
  G/RConn1 -- Component1_1_RIGID/RConn1
  Conn1/RConn1 -- Hip Pitch Joint/LConn1
  Knee Pitch Joint/RConn1 -- Component1_1_RIGID/LConn1
  Back Left Leg/RConn1 -- Hip Pitch Joint/RConn1
  Back Left Leg/LConn1 -- Knee Pitch Joint/LConn1

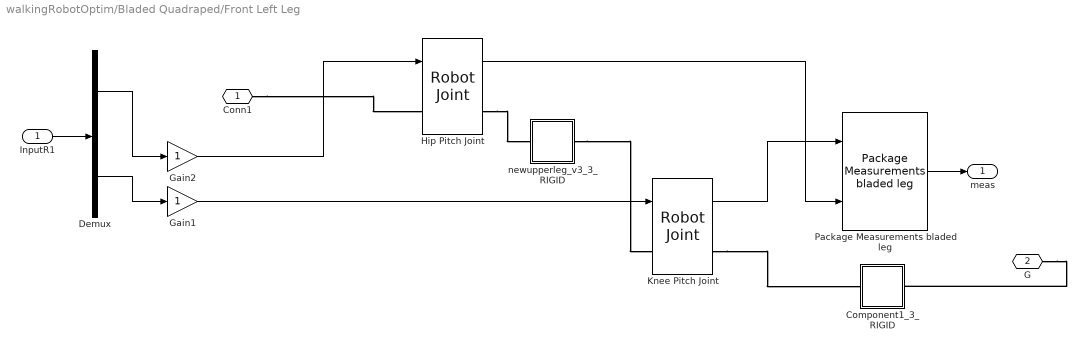
== system walkingRobotOptim/Bladed Quadraped/Front Left Leg ==
  InputR1 : Inport
  Component1_3_RIGID : Subsystem
  Demux : Demux  Outputs=2
  Gain1 : Gain
  Gain2 : Gain
  Hip Pitch Joint : walkingRobotUtils/Robot Joint  jointDamping=joint_damping  initAngle=init_angs_R(3)  upperLimit=pi/2  lowerLimit=-pi/2  limitK=1000  limitD=100
  Knee Pitch Joint : walkingRobotUtils/Robot Joint  jointDamping=joint_damping  initAngle=init_angs_R(5)  upperLimit=pi/2  lowerLimit=-pi/2  limitK=1000  limitD=100
  Package Measurements bladed leg : walkingRobotUtils/Package Measurements bladed leg  SystemSampleTime=-1  VariantActivationTime=update diagram  AllowFlexibleInterface=on  Latency=0  AutoFrameSizeCalculation=off
  newupperleg_v3_3_RIGID : Subsystem
  Conn1 : PMIOPort  Side=Left
  G : PMIOPort  Port=2  Side=Right
  meas : Outport  VectorParamsAs1DForOutWhenUnconnected=off
  wires:
  InputR1/1 -> Demux/1
  Demux/1 -> Gain2/1
  Demux/2 -> Gain1/1
  Gain2/1 -> Hip Pitch Joint/1
  Gain1/1 -> Knee Pitch Joint/1
  Hip Pitch Joint/1 -> Package Measurements bladed leg/2
  Knee Pitch Joint/1 -> Package Measurements bladed leg/1
  Package Measurements bladed leg/1 -> meas/1
  connections:
  G/RConn1 -- Component1_3_RIGID/RConn1
  Knee Pitch Joint/RConn1 -- Component1_3_RIGID/LConn1
  Conn1/RConn1 -- Hip Pitch Joint/LConn1
  Hip Pitch Joint/RConn1 -- newupperleg_v3_3_RIGID/LConn1
  newupperleg_v3_3_RIGID/RConn1 -- Knee Pitch Joint/LConn1

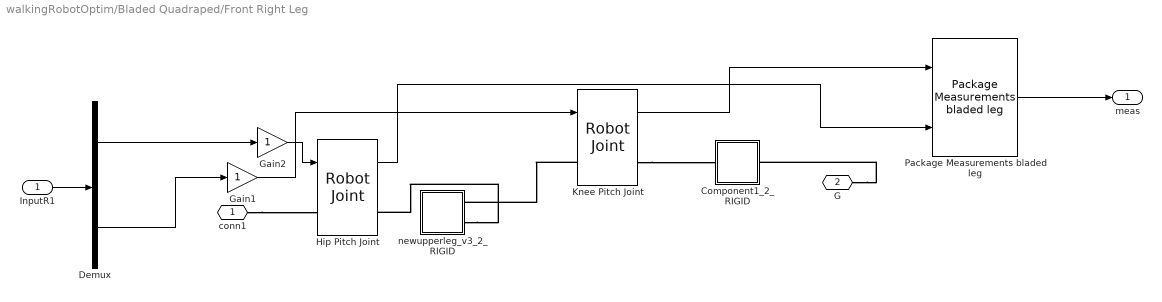
== system walkingRobotOptim/Bladed Quadraped/Front Right Leg ==
  InputR1 : Inport
  Component1_2_RIGID : Subsystem
  Demux : Demux  Outputs=2
  Gain1 : Gain
  Gain2 : Gain
  Hip Pitch Joint : walkingRobotUtils/Robot Joint  jointDamping=joint_damping  initAngle=init_angs_HR(1)  upperLimit=pi/2  lowerLimit=-pi/2  limitK=1000  limitD=100
  Knee Pitch Joint : walkingRobotUtils/Robot Joint  jointDamping=joint_damping  initAngle=init_angs_HR(2)  upperLimit=pi/2  lowerLimit=-pi/2  limitK=1000  limitD=100
  Package Measurements bladed leg : walkingRobotUtils/Package Measurements bladed leg  SystemSampleTime=-1  VariantActivationTime=update diagram  AllowFlexibleInterface=on  Latency=0  AutoFrameSizeCalculation=off
  newupperleg_v3_2_RIGID : Subsystem
  conn1 : PMIOPort  Side=Left
  G : PMIOPort  Port=2  Side=Right
  meas : Outport  VectorParamsAs1DForOutWhenUnconnected=off
  wires:
  Demux/2 -> Gain1/1
  InputR1/1 -> Demux/1
  Demux/1 -> Gain2/1
  Knee Pitch Joint/1 -> Package Measurements bladed leg/1
  Hip Pitch Joint/1 -> Package Measurements bladed leg/2
  Package Measurements bladed leg/1 -> meas/1
  Gain1/1 -> Knee Pitch Joint/1
  Gain2/1 -> Hip Pitch Joint/1
  connections:
  G/RConn1 -- Component1_2_RIGID/RConn1
  Knee Pitch Joint/RConn1 -- Component1_2_RIGID/LConn1
  Knee Pitch Joint/LConn1 -- newupperleg_v3_2_RIGID/RConn1
  conn1/RConn1 -- Hip Pitch Joint/LConn1
  newupperleg_v3_2_RIGID/RConn2 -- Hip Pitch Joint/RConn1

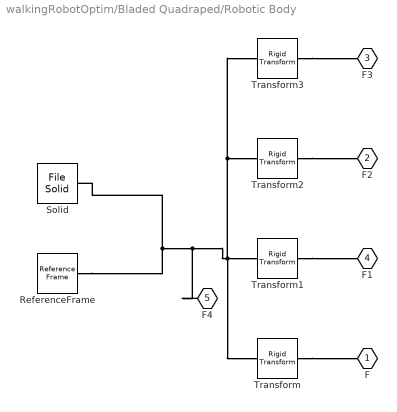
== system walkingRobotOptim/Bladed Quadraped/Robotic Body ==
  ReferenceFrame : sm_lib/Frames and Transforms/Reference Frame
  Solid : sm_lib/Body Elements/File Solid  ExtGeomFileName=robobody v1.step  UnitType=FromFile  ExtGeomFileUnits=m  StepReaderType=HEX  ExportConvexHullGeometry=off  InertiaType=CalculateFromGeometry  BasedOnType=Mass  Density=1000  DensityUnits=kg/m^3  Mass=body_weight  MassUnits=kg  CenterOfMass=smiData.Solid(3).CoM  CenterOfMassUnits=mm  MomentsOfInertia=smiData.Solid(3).MoI  MomentsOfInertiaUnits=lbm*mm^2  ProductsOfInertia=smiData.Solid(3).PoI  ProductsOfInertiaUnits=lbm*mm^2  GraphicType=FromGeometry  MarkerShape=Sphere  MarkerSize=10  GraphicVisPropType=SimpleVisualProperties  GraphicDiffuseColor=smiData.Solid(3).color  GraphicOpacity=smiData.Solid(3).opacity  GraphicSpecularColor=[0.5 0.5 0.5 1.0]  GraphicAmbientColor=[0.15 0.15 0.15 1.0]  GraphicEmissiveColor=[0.0 0.0 0.0 1.0]  GraphicShininess=75  DoExposeReferenceFrame=on  SerializedFrames=<Frames/>
  Transform : sm_lib/Frames and Transforms/Rigid Transform  RotationMethod=ArbitraryAxis  FollAlignAxisA=+X  BaseAlignAxisA=+Y  FollAlignAxisB=+Y  BaseAlignAxisB=+Z  RotationStandardAxis=+Z  RotationAngle=smiData.RigidTransform(2).angle  RotationAngleUnits=rad  RotationArbitraryAxis=smiData.RigidTransform(2).axis  RotationSequenceAxes=FollowerAxes  RotationSequence=XYX  RotationSequenceAngles=[0 0 0]  RotationSequenceAnglesUnits=deg  RotationMatrix=[1 0 0;0 1 0;0 0 1]  Quaternion=[1 0 0 0]  TranslationMethod=Cartesian  TranslationCartesianOffset=smiData.RigidTransform(2).translation  TranslationCartesianOffsetUnits=mm  TranslationStandardAxis=+Z  TranslationStandardOffset=0  TranslationStandardOffsetUnits=m  TranslationROffset=0  TranslationROffsetUnits=m  TranslationThetaOffset=0  TranslationThetaOffsetUnits=deg  TranslationZOffset=0  TranslationZOffsetUnits=m
  Transform1 : sm_lib/Frames and Transforms/Rigid Transform  RotationMethod=ArbitraryAxis  FollAlignAxisA=+X  BaseAlignAxisA=+Y  FollAlignAxisB=+Y  BaseAlignAxisB=+Z  RotationStandardAxis=+Z  RotationAngle=smiData.RigidTransform(7).angle  RotationAngleUnits=rad  RotationArbitraryAxis=smiData.RigidTransform(7).axis  RotationSequenceAxes=FollowerAxes  RotationSequence=XYX  RotationSequenceAngles=[0 0 0]  RotationSequenceAnglesUnits=deg  RotationMatrix=[1 0 0;0 1 0;0 0 1]  Quaternion=[1 0 0 0]  TranslationMethod=Cartesian  TranslationCartesianOffset=smiData.RigidTransform(7).translation  TranslationCartesianOffsetUnits=mm  TranslationStandardAxis=+Z  TranslationStandardOffset=0  TranslationStandardOffsetUnits=m  TranslationROffset=0  TranslationROffsetUnits=m  TranslationThetaOffset=0  TranslationThetaOffsetUnits=deg  TranslationZOffset=0  TranslationZOffsetUnits=m
  Transform2 : sm_lib/Frames and Transforms/Rigid Transform  RotationMethod=ArbitraryAxis  FollAlignAxisA=+X  BaseAlignAxisA=+Y  FollAlignAxisB=+Y  BaseAlignAxisB=+Z  RotationStandardAxis=+Z  RotationAngle=smiData.RigidTransform(10).angle  RotationAngleUnits=rad  RotationArbitraryAxis=smiData.RigidTransform(10).axis  RotationSequenceAxes=FollowerAxes  RotationSequence=XYX  RotationSequenceAngles=[0 0 0]  RotationSequenceAnglesUnits=deg  RotationMatrix=[1 0 0;0 1 0;0 0 1]  Quaternion=[1 0 0 0]  TranslationMethod=Cartesian  TranslationCartesianOffset=smiData.RigidTransform(10).translation  TranslationCartesianOffsetUnits=mm  TranslationStandardAxis=+Z  TranslationStandardOffset=0  TranslationStandardOffsetUnits=m  TranslationROffset=0  TranslationROffsetUnits=m  TranslationThetaOffset=0  TranslationThetaOffsetUnits=deg  TranslationZOffset=0  TranslationZOffsetUnits=m
  Transform3 : sm_lib/Frames and Transforms/Rigid Transform  RotationMethod=ArbitraryAxis  FollAlignAxisA=+X  BaseAlignAxisA=+Y  FollAlignAxisB=+Y  BaseAlignAxisB=+Z  RotationStandardAxis=+Z  RotationAngle=smiData.RigidTransform(11).angle  RotationAngleUnits=rad  RotationArbitraryAxis=smiData.RigidTransform(11).axis  RotationSequenceAxes=FollowerAxes  RotationSequence=XYX  RotationSequenceAngles=[0 0 0]  RotationSequenceAnglesUnits=deg  RotationMatrix=[1 0 0;0 1 0;0 0 1]  Quaternion=[1 0 0 0]  TranslationMethod=Cartesian  TranslationCartesianOffset=smiData.RigidTransform(11).translation  TranslationCartesianOffsetUnits=mm  TranslationStandardAxis=+Z  TranslationStandardOffset=0  TranslationStandardOffsetUnits=m  TranslationROffset=0  TranslationROffsetUnits=m  TranslationThetaOffset=0  TranslationThetaOffsetUnits=deg  TranslationZOffset=0  TranslationZOffsetUnits=m
  F : PMIOPort  Side=Left
  F2 : PMIOPort  Port=2  Side=Left
  F3 : PMIOPort  Port=3  Side=Right
  F1 : PMIOPort  Port=4  Side=Right
  F4 : PMIOPort  Port=5  Side=Right
  connections:
  Solid/RConn1 -- F4/RConn1 -- Transform2/LConn1 -- Transform3/LConn1 -- Transform/LConn1 -- Transform1/LConn1 -- ReferenceFrame/RConn1
  Transform/RConn1 -- F/RConn1
  Transform1/RConn1 -- F1/RConn1
  Transform2/RConn1 -- F2/RConn1
  Transform3/RConn1 -- F3/RConn1

== system walkingRobotOptim/Evaluate Joint Trajectories (Fore)/Create Bus L ==
  vec : Inport
  Bus Creator : BusCreator  Inputs=2
  Demux : Demux  Outputs=2
  Gain : Gain  Gain=-1
  bus : Outport  VectorParamsAs1DForOutWhenUnconnected=off
  wires:
  Demux/1 -> Bus Creator/1  "hip pitch"
  Gain/1 -> Demux/1
  Bus Creator/1 -> bus/1
  Demux/2 -> Bus Creator/2  "knee"
  vec/1 -> Gain/1

== system walkingRobotOptim/Evaluate Joint Trajectories (Fore)/Create Bus R1 ==
  vec : Inport
  Bus Creator : BusCreator  Inputs=2
  Demux : Demux  Outputs=2
  Gain : Gain  Gain=-1
  bus : Outport  VectorParamsAs1DForOutWhenUnconnected=off
  wires:
  Bus Creator/1 -> bus/1
  vec/1 -> Gain/1
  Demux/2 -> Bus Creator/2  "knee"
  Demux/1 -> Bus Creator/1  "hip pitch"
  Gain/1 -> Demux/1

== system walkingRobotOptim/Evaluate Joint Trajectories (Hind)/Create Bus L ==
  vec : Inport
  Bus Creator : BusCreator  Inputs=2
  Demux : Demux  Outputs=2
  Gain : Gain  Gain=-1
  bus : Outport  VectorParamsAs1DForOutWhenUnconnected=off
  wires:
  Demux/1 -> Bus Creator/1  "hip pitch"
  Gain/1 -> Demux/1
  Bus Creator/1 -> bus/1
  Demux/2 -> Bus Creator/2  "knee"
  vec/1 -> Gain/1

== system walkingRobotOptim/Evaluate Joint Trajectories (Hind)/Create Bus R1 ==
  vec : Inport
  Bus Creator : BusCreator  Inputs=2
  Demux : Demux  Outputs=2
  Gain : Gain  Gain=-1
  bus : Outport  VectorParamsAs1DForOutWhenUnconnected=off
  wires:
  Bus Creator/1 -> bus/1
  vec/1 -> Gain/1
  Demux/2 -> Bus Creator/2  "knee"
  Demux/1 -> Bus Creator/1  "hip pitch"
  Gain/1 -> Demux/1

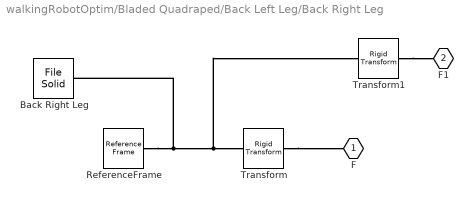
== system walkingRobotOptim/Bladed Quadraped/Back Left Leg/Back Right Leg ==
  Back Right Leg : sm_lib/Body Elements/File Solid  ExtGeomFileName=newupperleg v3.step  UnitType=FromFile  ExtGeomFileUnits=m  StepReaderType=HEX  ExportConvexHullGeometry=off  InertiaType=CalculateFromGeometry  BasedOnType=Mass  Density=1000  DensityUnits=kg/m^3  Mass=back_leg_weight  MassUnits=kg  CenterOfMass=smiData.Solid(1).CoM  CenterOfMassUnits=mm  MomentsOfInertia=smiData.Solid(1).MoI  MomentsOfInertiaUnits=lbm*mm^2  ProductsOfInertia=smiData.Solid(1).PoI  ProductsOfInertiaUnits=lbm*mm^2  GraphicType=FromGeometry  MarkerShape=Sphere  MarkerSize=10  GraphicVisPropType=SimpleVisualProperties  GraphicDiffuseColor=[0 0.4471 0.7412]  GraphicOpacity=smiData.Solid(1).opacity  GraphicSpecularColor=[0.5 0.5 0.5 1.0]  GraphicAmbientColor=[0.15 0.15 0.15 1.0]  GraphicEmissiveColor=[0.0 0.0 0.0 1.0]  GraphicShininess=75  DoExposeReferenceFrame=on  SerializedFrames=<Frames/>
  ReferenceFrame : sm_lib/Frames and Transforms/Reference Frame
  Transform : sm_lib/Frames and Transforms/Rigid Transform  RotationMethod=ArbitraryAxis  FollAlignAxisA=+X  BaseAlignAxisA=+Y  FollAlignAxisB=+Y  BaseAlignAxisB=+Z  RotationStandardAxis=+Z  RotationAngle=smiData.RigidTransform(8).angle  RotationAngleUnits=rad  RotationArbitraryAxis=smiData.RigidTransform(8).axis  RotationSequenceAxes=FollowerAxes  RotationSequence=XYX  RotationSequenceAngles=[0 0 0]  RotationSequenceAnglesUnits=deg  RotationMatrix=[1 0 0;0 1 0;0 0 1]  Quaternion=[1 0 0 0]  TranslationMethod=Cartesian  TranslationCartesianOffset=smiData.RigidTransform(8).translation  TranslationCartesianOffsetUnits=mm  TranslationStandardAxis=+Z  TranslationStandardOffset=0  TranslationStandardOffsetUnits=m  TranslationROffset=0  TranslationROffsetUnits=m  TranslationThetaOffset=0  TranslationThetaOffsetUnits=deg  TranslationZOffset=0  TranslationZOffsetUnits=m
  Transform1 : sm_lib/Frames and Transforms/Rigid Transform  RotationMethod=ArbitraryAxis  FollAlignAxisA=+X  BaseAlignAxisA=+Y  FollAlignAxisB=+Y  BaseAlignAxisB=+Z  RotationStandardAxis=+Z  RotationAngle=smiData.RigidTransform(13).angle  RotationAngleUnits=rad  RotationArbitraryAxis=smiData.RigidTransform(13).axis  RotationSequenceAxes=FollowerAxes  RotationSequence=XYX  RotationSequenceAngles=[0 0 0]  RotationSequenceAnglesUnits=deg  RotationMatrix=[1 0 0;0 1 0;0 0 1]  Quaternion=[1 0 0 0]  TranslationMethod=Cartesian  TranslationCartesianOffset=smiData.RigidTransform(13).translation  TranslationCartesianOffsetUnits=mm  TranslationStandardAxis=+Z  TranslationStandardOffset=0  TranslationStandardOffsetUnits=m  TranslationROffset=0  TranslationROffsetUnits=m  TranslationThetaOffset=0  TranslationThetaOffsetUnits=deg  TranslationZOffset=0  TranslationZOffsetUnits=m
  F : PMIOPort  Side=Left
  F1 : PMIOPort  Port=2  Side=Right
  connections:
  Back Right Leg/RConn1 -- Transform/LConn1 -- Transform1/LConn1 -- ReferenceFrame/RConn1
  Transform/RConn1 -- F/RConn1
  Transform1/RConn1 -- F1/RConn1

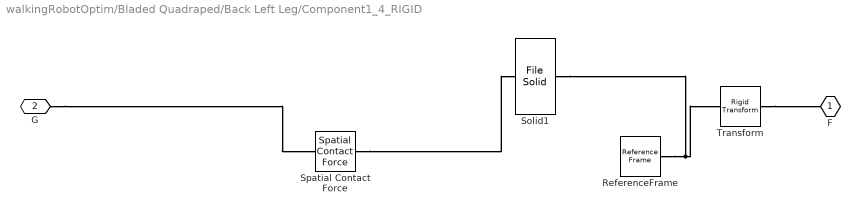
== system walkingRobotOptim/Bladed Quadraped/Back Left Leg/Component1_4_RIGID ==
  ReferenceFrame : sm_lib/Frames and Transforms/Reference Frame
  Solid1 : sm_lib/Body Elements/File Solid  ExtGeomFileName=Component1.step  UnitType=FromFile  ExtGeomFileUnits=m  StepReaderType=HEX  ExportConvexHullGeometry=on  InertiaType=CalculateFromGeometry  BasedOnType=Mass  Density=1000  DensityUnits=kg/m^3  Mass=half_leg_weight  MassUnits=kg  CenterOfMass=smiData.Solid(2).CoM  CenterOfMassUnits=mm  MomentsOfInertia=smiData.Solid(2).MoI  MomentsOfInertiaUnits=lbm*mm^2  ProductsOfInertia=smiData.Solid(2).PoI  ProductsOfInertiaUnits=lbm*mm^2  GraphicType=FromGeometry  MarkerShape=Sphere  MarkerSize=10  GraphicVisPropType=SimpleVisualProperties  GraphicDiffuseColor=smiData.Solid(2).color  GraphicOpacity=smiData.Solid(2).opacity  GraphicSpecularColor=[0.5 0.5 0.5 1.0]  GraphicAmbientColor=[0.15 0.15 0.15 1.0]  GraphicEmissiveColor=[0.0 0.0 0.0 1.0]  GraphicShininess=75  DoExposeReferenceFrame=on  SerializedFrames=<Frames/>
  Spatial Contact Force : sm_lib/Forces and Torques/Spatial Contact Force  NormalForceType=SmoothSpringDamper  NormalStiffness=1e6  NormalStiffnessUnits=N/m  NormalDamping=1e3  NormalDampingUnits=N/(m/s)  NormalTransitionRegionWidth=1e-4  NormalTransitionRegionWidthUnits=m  FrictionType=SmoothStickSlip  CoefficientOfStaticFriction=friction_coefficient  CoefficientOfDynamicFriction=friction_coefficient  FrictionalCriticalVelocity=1e-3  FrictionalCriticalVelocityUnits=m/s  SenseContactSignal=off  SensePenetrationDepth=off  SenseSeparationDistance=off  SenseNormalForceMagnitude=off  SenseFrictionalForceMagnitude=off  SenseNormalVelocity=off  SenseTangentialVelocity=off  SenseContactBaseRotation=off  SenseContactBaseTranslation=off  SenseContactFollowerRotation=off  SenseContactFollowerTranslation=off  ZeroCrossDetectContactStartAndEnd=off
  Transform : sm_lib/Frames and Transforms/Rigid Transform  RotationMethod=ArbitraryAxis  FollAlignAxisA=+X  BaseAlignAxisA=+Y  FollAlignAxisB=+Y  BaseAlignAxisB=+Z  RotationStandardAxis=+Z  RotationAngle=smiData.RigidTransform(14).angle  RotationAngleUnits=rad  RotationArbitraryAxis=smiData.RigidTransform(14).axis  RotationSequenceAxes=FollowerAxes  RotationSequence=XYX  RotationSequenceAngles=[0 0 0]  RotationSequenceAnglesUnits=deg  RotationMatrix=[1 0 0;0 1 0;0 0 1]  Quaternion=[1 0 0 0]  TranslationMethod=Cartesian  TranslationCartesianOffset=smiData.RigidTransform(14).translation  TranslationCartesianOffsetUnits=mm  TranslationStandardAxis=+Z  TranslationStandardOffset=0  TranslationStandardOffsetUnits=m  TranslationROffset=0  TranslationROffsetUnits=m  TranslationThetaOffset=0  TranslationThetaOffsetUnits=deg  TranslationZOffset=0  TranslationZOffsetUnits=m
  F : PMIOPort  Side=Left
  G : PMIOPort  Port=2  Side=Right
  connections:
  ReferenceFrame/RConn1 -- Solid1/RConn1 -- Transform/LConn1
  Transform/RConn1 -- F/RConn1
  Spatial Contact Force/RConn1 -- Solid1/LConn1
  G/RConn1 -- Spatial Contact Force/LConn1

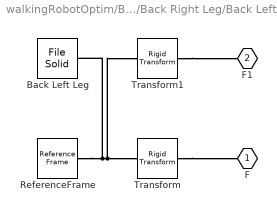
== system walkingRobotOptim/Bladed Quadraped/Back Right Leg/Back Left Leg ==
  Back Left Leg : sm_lib/Body Elements/File Solid  ExtGeomFileName=newupperleg v3.step  UnitType=FromFile  ExtGeomFileUnits=m  StepReaderType=HEX  ExportConvexHullGeometry=off  InertiaType=CalculateFromGeometry  BasedOnType=Mass  Density=1000  DensityUnits=kg/m^3  Mass=back_leg_weight  MassUnits=kg  CenterOfMass=smiData.Solid(1).CoM  CenterOfMassUnits=mm  MomentsOfInertia=smiData.Solid(1).MoI  MomentsOfInertiaUnits=lbm*mm^2  ProductsOfInertia=smiData.Solid(1).PoI  ProductsOfInertiaUnits=lbm*mm^2  GraphicType=FromGeometry  MarkerShape=Sphere  MarkerSize=10  GraphicVisPropType=SimpleVisualProperties  GraphicDiffuseColor=[1 0 1]  GraphicOpacity=smiData.Solid(1).opacity  GraphicSpecularColor=[0.5 0.5 0.5 1.0]  GraphicAmbientColor=[0.15 0.15 0.15 1.0]  GraphicEmissiveColor=[0.0 0.0 0.0 1.0]  GraphicShininess=75  DoExposeReferenceFrame=on  SerializedFrames=<Frames/>
  ReferenceFrame : sm_lib/Frames and Transforms/Reference Frame
  Transform : sm_lib/Frames and Transforms/Rigid Transform  RotationMethod=ArbitraryAxis  FollAlignAxisA=+X  BaseAlignAxisA=+Y  FollAlignAxisB=+Y  BaseAlignAxisB=+Z  RotationStandardAxis=+Z  RotationAngle=smiData.RigidTransform(5).angle  RotationAngleUnits=rad  RotationArbitraryAxis=smiData.RigidTransform(5).axis  RotationSequenceAxes=FollowerAxes  RotationSequence=XYX  RotationSequenceAngles=[0 0 0]  RotationSequenceAnglesUnits=deg  RotationMatrix=[1 0 0;0 1 0;0 0 1]  Quaternion=[1 0 0 0]  TranslationMethod=Cartesian  TranslationCartesianOffset=smiData.RigidTransform(5).translation  TranslationCartesianOffsetUnits=mm  TranslationStandardAxis=+Z  TranslationStandardOffset=0  TranslationStandardOffsetUnits=m  TranslationROffset=0  TranslationROffsetUnits=m  TranslationThetaOffset=0  TranslationThetaOffsetUnits=deg  TranslationZOffset=0  TranslationZOffsetUnits=m
  Transform1 : sm_lib/Frames and Transforms/Rigid Transform  RotationMethod=ArbitraryAxis  FollAlignAxisA=+X  BaseAlignAxisA=+Y  FollAlignAxisB=+Y  BaseAlignAxisB=+Z  RotationStandardAxis=+Z  RotationAngle=smiData.RigidTransform(9).angle  RotationAngleUnits=rad  RotationArbitraryAxis=smiData.RigidTransform(9).axis  RotationSequenceAxes=FollowerAxes  RotationSequence=XYX  RotationSequenceAngles=[0 0 0]  RotationSequenceAnglesUnits=deg  RotationMatrix=[1 0 0;0 1 0;0 0 1]  Quaternion=[1 0 0 0]  TranslationMethod=Cartesian  TranslationCartesianOffset=smiData.RigidTransform(9).translation  TranslationCartesianOffsetUnits=mm  TranslationStandardAxis=+Z  TranslationStandardOffset=0  TranslationStandardOffsetUnits=m  TranslationROffset=0  TranslationROffsetUnits=m  TranslationThetaOffset=0  TranslationThetaOffsetUnits=deg  TranslationZOffset=0  TranslationZOffsetUnits=m
  F : PMIOPort  Side=Left
  F1 : PMIOPort  Port=2  Side=Right
  connections:
  Back Left Leg/RConn1 -- ReferenceFrame/RConn1 -- Transform/LConn1 -- Transform1/LConn1
  Transform/RConn1 -- F/RConn1
  Transform1/RConn1 -- F1/RConn1
